simulink model "test_ALSA"  (R2023a)
settings: Solver=FixedStepAuto  StartTime=0.0  StopTime=inf  RelTol=1e-3  EnableMultiTasking=on
InitFcn:
  | timespan=1;
  | sampling_subsample=2;
undefined symbols (not defined in the file or in its folder): plughw
libraries: raspberrypiAVlib x1, dspvision x1
settings Model: SimulationMode=external  ExtModeTrigDuration=2  Creator=tokamoto  LastModifiedBy=tokamoto
settings SolverCC: AlgebraicLoopSolver=TrustRegion  PositivePriorityOrder=on
settings DataIOCC: LimitDataPoints=on  DSMLogging=off  StreamToWks=off  ReturnWorkspaceOutputs=off
settings OptimizationCC: ZeroExternalMemoryAtStartup=off  ZeroInternalMemoryAtStartup=off  MaxStackSize=64
settings DebuggingCC: ParameterTunabilityLossMsg=error  UnconnectedInputMsg=warning  UnconnectedOutputMsg=warning  UnconnectedLineMsg=warning  ArithmeticOperatorsInVariantConditions=warning
settings HardwareCC: ProdBitPerLong=64  ProdLargestAtomicInteger=LongLong  ProdLargestAtomicFloat=Double  ProdLongLongMode=on  ProdHWDeviceType=ARM Compatible->ARM 64-bit (LP64)
settings ModelReferenceCC: EnableRefExpFcnMdlSchedulingChecks=on
settings SFSimCC: SimUseLocalCustomCode=off  CustomCodeUndefinedFunction=UseInterfaceOnly
settings RTWCC: Description=Embedded Coder  SystemTargetFile=ert.tlc  HardwareBoard=Raspberry Pi (64bit)  TemplateMakefile=ert_default_tmf  GenerateReport=on  RTWUseLocalCustomCode=off  Toolchain=GNU GCC Embedded Linux  BuildConfiguration=Faster Runs  LaunchReport=on  GenerateCodeMetricsReport=on
settings CodeAppCC: ForceParamTrailComments=on  OperatorAnnotations=on  StateflowObjectComments=on  MATLABSourceComments=on
settings ERTTargetCC: TargetLangStandard=C99 (ISO)  ERTCustomFileBanners=off  SupportContinuousTime=on  SupportNonInlinedSFcns=on  RemoveResetFunc=off  SupportVariableSizeSignals=on  ModelStepFunctionPrototypeControlCompliant=off  ExtMode=on  ExtModeTransport=2  ExtModeStaticAlloc=on  ExtModeMaxTrigDuration=1000  ExtModeMexFile=ext_xcp  ExtModeMexArgs='192.168.1.23' 0 17725  ExtModeIntrfLevel=Level2 - Open  RootIOFormat=Structure reference

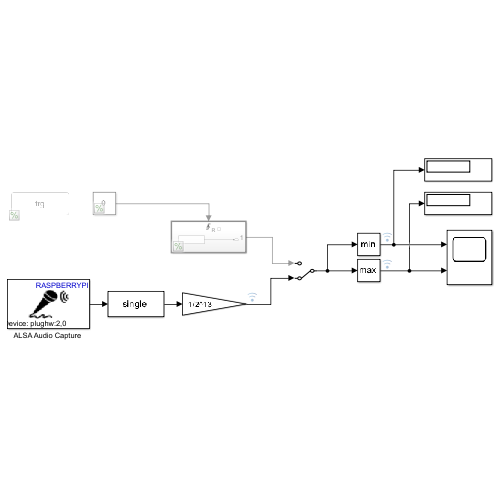
[thumbnail: Simulink's stored preview of the top-level diagram]
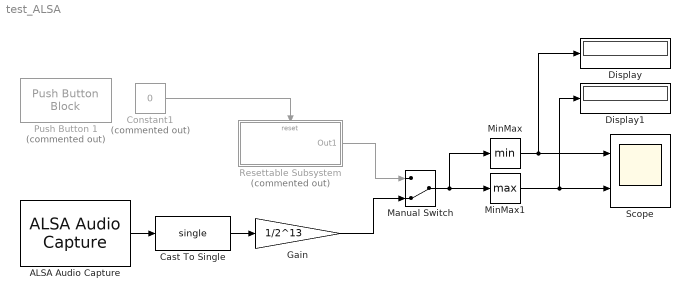
== system test_ALSA ==
  "ALSA Audio Capture " : raspberrypiAVlib/ALSA Audio Capture  deviceStr=plughw:2,0  DataBitDepth=16-bit integer  numberOfChannels=1  sampleRateEnum=44100  frameSize=441  QueueDuration=0.5  blockPlatform=LINUX
  Cast To Single : DataTypeConversion  OutDataTypeStr=single  SaturateOnIntegerOverflow=off  RndMeth=Floor
  Constant1 : Constant  Commented=on  Value=0
  Display : Display
  Display1 : Display
  Gain : Gain  Gain=1/2^13
  Manual Switch : ManualSwitch  CurrentSetting=0
  MinMax : MinMax
  MinMax1 : MinMax  Function=max
  Push Button 1 : PushButtonBlock  Commented=on  ButtonText=trg  OffValue=0.000000
  Resettable Subsystem : Subsystem  Commented=on  TreatAsAtomicUnit=on
  Scope : Scope  NumInputPorts=2
  wires:
  "ALSA Audio Capture "/1 -> Cast To Single/1
  Resettable Subsystem/1(Out1) -> Manual Switch/1
  Manual Switch/1 -> MinMax/1, MinMax1/1
  Constant1/1 -> Resettable Subsystem/Reset
  MinMax/1 -> Display/1, Scope/1
  MinMax1/1 -> Scope/2, Display1/1
  Gain/1 -> Manual Switch/2
  Cast To Single/1 -> Gain/1

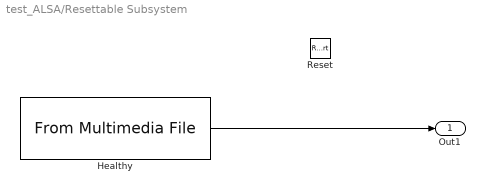
== system test_ALSA/Resettable Subsystem ==
  Reset : ResetPort  DisableCoverage=on
  Healthy : dspvision/From Multimedia File  inputFilename=C:\Users\tokamoto\MATLAB\Projects\Raspi\LSTM_Wavelet_HW\AirCompressorDataset\Healthy\preprocess_Reading2.wav  readRange=[1 inf]  loop=on  numPlays=1  outputStreams=オーディオのみ  videoDataType=single  audioDataType=double  inheritSampleTime=on  userDefinedSampleTime=1/16  noAudioOutput=off  isIntensityVideo=off  fourcc=RGB  colorVideoFormat=Separate color signals  outputEOF=off  dataOrg=Column-major  audioFrameSize=441  computeAudioFrameSize=off  outSamplingMode=Sample based
  Out1 : Outport
  wires:
  Healthy/1 -> Out1/1
